simulink model "Model_posCTRL_SS_2019a_1"  (R2022b)
settings: Solver=ode45  StartTime=0.0  StopTime=10  RelTol=1e-3
values from neighbouring files (symbols this model uses):
  A = [      0       1        0        0 ... (first row only)    [Code_od_2_axis _manipulator.m]    (also in skeleton_Open_loop_Model.m)
  B = [ 0 ... (first row only)    [Code_od_2_axis _manipulator.m]    (also in skeleton_Open_loop_Model.m)
  C = [ 0 0 1 0 ... (first row only)    [Code_od_2_axis _manipulator.m]    (also in skeleton_Open_loop_Model.m)
  D = [0;0]    [Code_od_2_axis _manipulator.m]    (also in skeleton_Open_loop_Model.m = [0;0;0])
  K_p_speed = 0.12    [Code_od_2_axis _manipulator.m]
  Kpos = 0.55    [Code_od_2_axis _manipulator.m]
  r = 0.032    [Code_od_2_axis _manipulator.m]    (also in skeleton_Open_loop_Model.m)
  Ti_speed = 3.5    [Code_od_2_axis _manipulator.m]
  Ts_pseudo = 1    [Code_od_2_axis _manipulator.m]
libraries: slpidlib x1
settings Model: Creator=lindh  LastModifiedBy=ficjuhu
settings SolverCC: AlgebraicLoopSolver=TrustRegion
settings DebuggingCC: UnconnectedInputMsg=warning  UnconnectedOutputMsg=warning  UnconnectedLineMsg=warning  SFMachineParentedDataDiag=warning
settings ModelReferenceCC: EnableRefExpFcnMdlSchedulingChecks=on
settings SFSimCC: CustomCodeUndefinedFunction=UseInterfaceOnly
settings RTWCC: DLArmComputeVersion=19.05

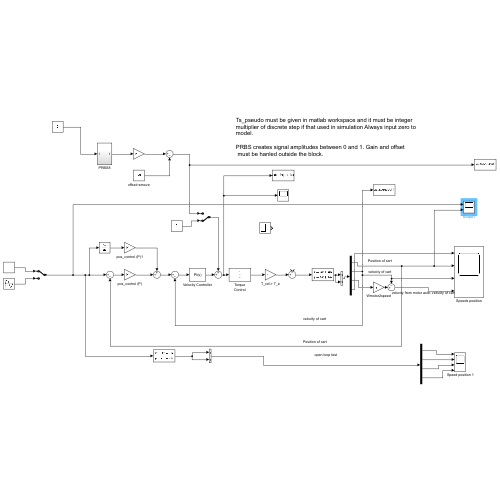
[thumbnail: Simulink's stored preview of the top-level diagram]
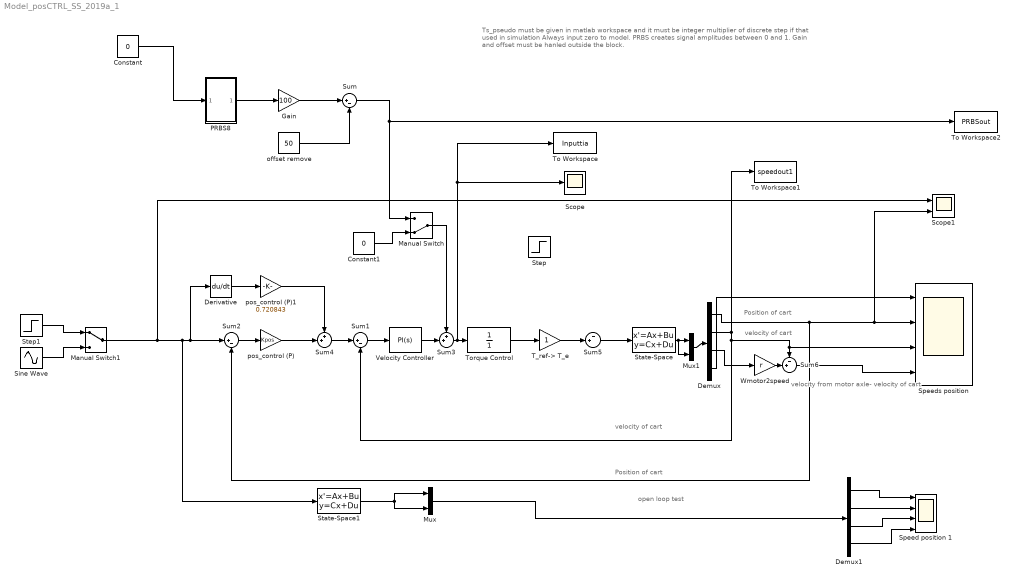
== system Model_posCTRL_SS_2019a_1 ==
  note: open loop test
  note: velocity from motor axle- velocity of cart
  note: velocity of cart
  note: Position of cart
  note: Ts_pseudo must be given in matlab workspace and it must be integer
      | multiplier of discrete step if that used in simulation Always input zero to
      | model.
      |
      | PRBS creates signal amplitudes between 0 and 1. Gain and offset
      | must be hanled outside the block.
  note: velocity of cart
  note: Position of cart
  " Speed position 1" : Scope  NumInputPorts=4
  " Speeds position " : Scope  NumInputPorts=4
  Constant : Constant  Value=0
  Constant1 : Constant  Value=0
  Demux : Demux
  Demux1 : Demux
  Derivative : Derivative
  Gain : Gain  Gain=100
  Manual Switch : ManualSwitch  CurrentSetting=0
  Manual Switch1 : ManualSwitch
  Mux : Mux  Inputs=2
      settings: DisplayOption=signals
  Mux1 : Mux  Inputs=2
      settings: DisplayOption=signals
  PRBS8 : Subsystem
  Scope : Scope
  Scope1 : Scope  NumInputPorts=2
  Sine Wave : Sin  Amplitude=0.5  Frequency=0.5  SampleTime=0
  State-Space : StateSpace  A=A  B=B  C=C  D=D  InitialCondition=0
  State-Space1 : StateSpace  A=A  B=B  C=C  D=D  InitialCondition=0
  Step : Step  Time=7  After=0.2  SampleTime=0
  Step1 : Step  SampleTime=0
  Sum : Sum  Inputs=|+-
  Sum1 : Sum  Inputs=|+-
  Sum2 : Sum  Inputs=|+-
  Sum3 : Sum  Inputs=++|
  Sum4 : Sum  Inputs=++|
  Sum5 : Sum  Inputs=-+|
  Sum6 : Sum  Inputs=-+|
  T_ref-> T_e : Gain
  To Workspace : ToWorkspace  VariableName=Inputtia  SampleTime=Ts_pseudo
  To Workspace1 : ToWorkspace  VariableName=speedout1  SampleTime=Ts_pseudo
  To Workspace2 : ToWorkspace  VariableName=PRBSout  SampleTime=Ts_pseudo
  Torque Control : TransferFcn  Numerator=1  Denominator=1
  Velocity Controller : slpidlib/PID Controller  Controller=PI  Form=Parallel  TimeDomain=Continuous-time  UseExternalTs=off  SampleTime=-1  IntegratorMethod=Forward Euler  FilterMethod=Forward Euler  ControllerParametersSource=internal  P=K_p_speed  I=Ti_speed  UseKiTs=off  D=-2.56884921321479  N=0.590053636621927  UseFilter=on  TunerSelectOption=Transfer Function Based (PID Tuner App)  InitialConditionSource=internal  InitialConditionForIntegrator=0  InitialConditionForFilter=0  DifferentiatorICPrevScaledInput=0  ExternalReset=none  TrackingMode=off  Kt=1  LimitOutput=off  SatLimitsSource=internal  UpperSaturationLimit=inf  LowerSaturationLimit=-inf  LinearizeAsGain=on  AntiWindupMode=none  Kb=1  LimitIntegrator=off  UpperIntegratorSaturationLimit=inf  LowerIntegratorSaturationLimit=-inf  POutMin=[]  POutMax=[]  IOutMin=[]  IOutMax=[]  DOutMin=[]  DOutMax=[]  NOutMin=[]  NOutMax=[]  SumOutMin=[]  SumOutMax=[]  SaturationOutMin=[]  SaturationOutMax=[]  PParamMin=[]  PParamMax=[]  IParamMin=[]  IParamMax=[]  DParamMin=[]  DParamMax=[]  NParamMin=[]  NParamMax=[]  KbParamMin=[]  KbParamMax=[]  KtParamMin=[]  KtParamMax=[]  KbOutMin=[]  KbOutMax=[]  KtOutMin=[]  KtOutMax=[]  IntegratorOutMin=[]  IntegratorOutMax=[]  FilterOutMin=[]  FilterOutMax=[]  SumI1OutMin=[]  SumI1OutMax=[]  SumI2OutMin=[]  SumI2OutMax=[]  SumI3OutMin=[]  SumI3OutMax=[]  SumI4OutMin=[]  SumI4OutMax=[]  SumDOutMin=[]  SumDOutMax=[]  DifferentiatorOutMin=[]  DifferentiatorOutMax=[]  FilterDiffOutCoefMin=[]  FilterDiffOutCoefMax=[]  ReciprocalOutMin=[]  ReciprocalOutMax=[]  SumDenOutMin=[]  SumDenOutMax=[]  SumNumOutMin=[]  SumNumOutMax=[]  DivideOutMin=[]  DivideOutMax=[]  UdiffTsProdOutMin=[]  UdiffTsProdOutMax=[]  NTsProdOutMin=[]  NTsProdOutMax=[]  UintegralTsProdOutMin=[]  UintegralTsProdOutMax=[]  UngainTsProdOutMin=[]  UngainTsProdOutMax=[]  ClampingZeroOutDataTypeStr=Inherit: Inherit via back propagation  ClampingZeroOutMin=[]  ClampingZeroOutMax=[]  FilterDenConstantOutDataTypeStr=Inherit: Inherit via back propagation  FilterDenConstantOutMin=[]  FilterDenConstantOutMax=[]  PCopyOutDataTypeStr=Inherit: Inherit via back propagation  PCopyOutMin=[]  PCopyOutMax=[]  NCopyOutDataTypeStr=Inherit: Inherit via back propagation  NCopyOutMin=[]  NCopyOutMax=[]  IntegratorContinuousStateAttributes=''  IntegratorStateMustResolveToSignalObject=off  IntegratorRTWStateStorageClass=Auto  FilterContinuousStateAttributes=''  FilterStateMustResolveToSignalObject=off  FilterRTWStateStorageClass=Auto  ParallelPVariant=InternalParameters  IdealPVariant=Disabled  IVariant=InternalParameters  DVariant=Disabled  IntegratorVariant=Continuous  SatVariant=Disabled  AWVariant=Passthrough  PCopyVariant=Disabled  TRVariant=Disabled  FdbkBlocksVariant=Forward  IdealPFdbkVariant=Disabled  SatFdbkVariant=Disabled  DerivativeFilterVariant=Disabled  NVariant=Disabled  NCopyVariant=Disabled_SignalSpec  FilterICVariant=Disabled  IntegratorICVariant=InternalICs  ExternalResetVariant=Disabled  TRSumVariant=Passthrough  SumFdbkVariant=Disabled  SumVariant=Sum_PI  TsampFilterVariant=InternalTs  TsampNgainVariant=Passthrough  TsampIntegralVariant=Passthrough  ExternalSaturationOutDataTypeStr=Inherit: Same as second input
  Wmotor2speed : Gain  Gain=r
  offset remove : Constant  Value=50
  pos_control (P) : Gain  Gain=Kpos
  pos_control (P)1 : Gain  Gain=0.720843
  wires:
  Sum2/1 -> pos_control (P)/1
  pos_control (P)/1 -> Sum4/2
  Manual Switch1/1 -> Scope1/1, State-Space1/1, Derivative/1, Sum2/1
  Sum4/1 -> Sum1/1
  pos_control (P)1/1 -> Sum4/1
  Derivative/1 -> pos_control (P)1/1
  Sum1/1 -> Velocity Controller/1
  Torque Control/1 -> T_ref-> T_e/1
  T_ref-> T_e/1 -> Sum5/2
  Velocity Controller/1 -> Sum3/2
  Sum3/1 -> Scope/1, To Workspace/1, Torque Control/1
  PRBS8/1(Out1) -> Gain/1
  offset remove/1 -> Sum/2
  Sum/1 -> To Workspace2/1, Manual Switch/1
  Gain/1 -> Sum/1
  Constant/1 -> PRBS8/1(In1)
  Constant1/1 -> Manual Switch/2
  Manual Switch/1 -> Sum3/1
  Sum5/1 -> State-Space/1
  Demux/3 -> Wmotor2speed/1
  Demux/1 -> Sum2/2, Scope1/2, " Speeds position "/2
  Demux/2 -> Sum1/2, Sum6/1, " Speeds position "/3, To Workspace1/1
  Wmotor2speed/1 -> Sum6/2
  Demux1/2 -> " Speed position 1"/2
  Demux1/1 -> " Speed position 1"/1
  State-Space1/1 -> Mux/2, Mux/1
  Sum6/1 -> " Speeds position "/4
  Mux/1 -> Demux1/1
  Demux1/3 -> " Speed position 1"/3
  Demux1/4 -> " Speed position 1"/4
  State-Space/1 -> Mux1/2, Mux1/1
  Mux1/1 -> Demux/1
  Demux/4 -> " Speeds position "/1
  Step1/1 -> Manual Switch1/1
  Sine Wave/1 -> Manual Switch1/2

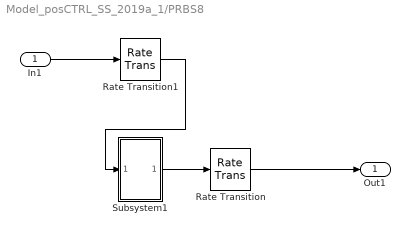
== system Model_posCTRL_SS_2019a_1/PRBS8 ==
  In1 : Inport
  Rate Transition : RateTransition  Deterministic=off  OutPortSampleTime=Ts_pseudo
  Rate Transition1 : RateTransition  OutPortSampleTime=Ts_pseudo
  Subsystem1 : Subsystem
  Out1 : Outport  VectorParamsAs1DForOutWhenUnconnected=off
  wires:
  Rate Transition1/1 -> Subsystem1/1(In1)
  Subsystem1/1(PRBS1) -> Rate Transition/1
  Rate Transition/1 -> Out1/1
  In1/1 -> Rate Transition1/1

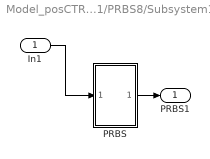
== system Model_posCTRL_SS_2019a_1/PRBS8/Subsystem1 ==
  In1 : Inport
  PRBS : Subsystem
  PRBS1 : Outport  VectorParamsAs1DForOutWhenUnconnected=off
  wires:
  PRBS/1(Out1) -> PRBS1/1
  In1/1 -> PRBS/1(In1)

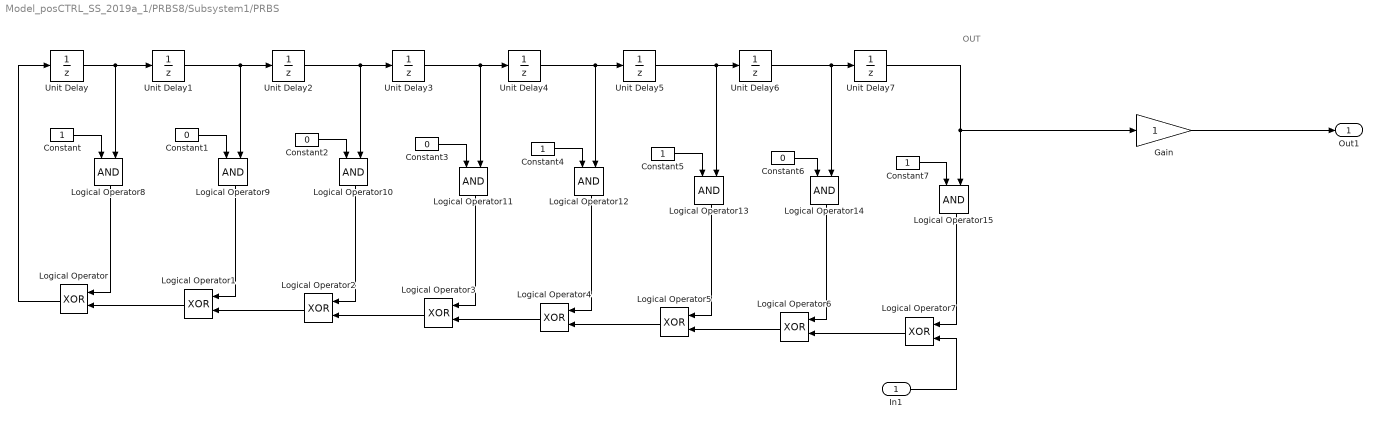
== system Model_posCTRL_SS_2019a_1/PRBS8/Subsystem1/PRBS ==
  note: OUT
  In1 : Inport
  Constant{,4..5,7} (4 alike) : Constant  OutDataTypeStr=boolean
  Constant{1..3,6} (4 alike) : Constant  Value=0  OutDataTypeStr=boolean
  Gain : Gain
  Logical Operator{,1..7} (8 alike) : Logic  Operator=XOR  AllPortsSameDT=off  OutDataTypeStr=boolean
  Logical Operator{8..15} (8 alike) : Logic  AllPortsSameDT=off  OutDataTypeStr=boolean
  Unit Delay{,1..7} (8 alike) : UnitDelay  InitialCondition=1  SampleTime=-1  HasFrameUpgradeWarning=on
  Out1 : Outport  VectorParamsAs1DForOutWhenUnconnected=off
  wires:
  Gain/1 -> Out1/1
  Logical Operator7/1 -> Logical Operator6/2
  Logical Operator15/1 -> Logical Operator7/1
  Constant7/1 -> Logical Operator15/1
  Logical Operator6/1 -> Logical Operator5/2
  Logical Operator14/1 -> Logical Operator6/1
  Constant6/1 -> Logical Operator14/1
  Logical Operator5/1 -> Logical Operator4/2
  Logical Operator13/1 -> Logical Operator5/1
  Constant5/1 -> Logical Operator13/1
  Logical Operator4/1 -> Logical Operator3/2
  Logical Operator12/1 -> Logical Operator4/1
  Constant4/1 -> Logical Operator12/1
  Logical Operator3/1 -> Logical Operator2/2
  Logical Operator11/1 -> Logical Operator3/1
  Constant3/1 -> Logical Operator11/1
  Logical Operator2/1 -> Logical Operator1/2
  Logical Operator10/1 -> Logical Operator2/1
  Constant2/1 -> Logical Operator10/1
  Logical Operator1/1 -> Logical Operator/2
  Logical Operator9/1 -> Logical Operator1/1
  Constant1/1 -> Logical Operator9/1
  Logical Operator8/1 -> Logical Operator/1
  Constant/1 -> Logical Operator8/1
  Logical Operator/1 -> Unit Delay/1
  Unit Delay7/1 -> Gain/1, Logical Operator15/2
  Unit Delay6/1 -> Unit Delay7/1, Logical Operator14/2
  Unit Delay5/1 -> Logical Operator13/2, Unit Delay6/1
  Unit Delay4/1 -> Logical Operator12/2, Unit Delay5/1
  Unit Delay3/1 -> Logical Operator11/2, Unit Delay4/1
  Unit Delay2/1 -> Logical Operator10/2, Unit Delay3/1
  Unit Delay1/1 -> Logical Operator9/2, Unit Delay2/1
  Unit Delay/1 -> Logical Operator8/2, Unit Delay1/1
  In1/1 -> Logical Operator7/2
